simulink model "Reto3"  (R2013a)
settings: Solver=ode45  StartTime=0.0  StopTime=4  RelTol=1e-3
settings Model: Creator=Henry Orlando  LastModifiedBy=Henry Orlando

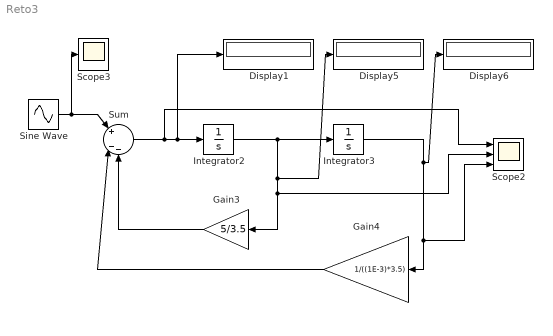
== system Reto3 ==
  Display1 : Display
  Display5 : Display
  Display6 : Display
  Gain3 : Gain  Gain=5/3.5
  Gain4 : Gain  Gain=1/((1E-3)*3.5)
  Integrator2 : Integrator
  Integrator3 : Integrator
  Scope2 : Scope  NumInputPorts=3
      settings: YMin=-5~-5~-5  YMax=5~5~5
  Scope3 : Scope
      settings: SaveName=ScopeData2
  Sine Wave : Sin  Amplitude=12/3.5  SampleTime=0
  Sum : Sum  Inputs=|+|--
  wires:
  Gain3/1 -> Sum/3
  Gain4/1 -> Sum/2
  Sine Wave/1 -> Scope3/1, Sum/1
  Sum/1 -> Scope2/1, Display1/1, Integrator2/1
  Integrator2/1 -> Integrator3/1, Display5/1, Scope2/2, Gain3/1
  Integrator3/1 -> Display6/1, Scope2/3, Gain4/1
